simulink model "Verkehrspolizist"  (Simulink 8.7)
settings: Solver=FixedStepAuto  StartTime=0.0  StopTime=10.0  FixedStep=0.01  RelTol=1e-3
settings Model: Creator=eispin  LastModifiedBy=max
settings DataIOCC: LimitDataPoints=off  SaveFormat=Dataset
settings DebuggingCC: UnderspecifiedInitializationDetection=Simplified  MergeDetectMultiDrivingBlocksExec=error
settings HardwareCC: ProdBitPerPointer=64  ProdLargestAtomicFloat=Float  ProdIntDivRoundTo=Zero  ProdEndianess=LittleEndian  ProdWordSize=64  ProdHWDeviceType=Intel->x86-64 (Windows64)
settings ModelReferenceCC: PropagateSignalLabelsOutOfModel=on
settings ConfigComp: CovModelRefEnable=off

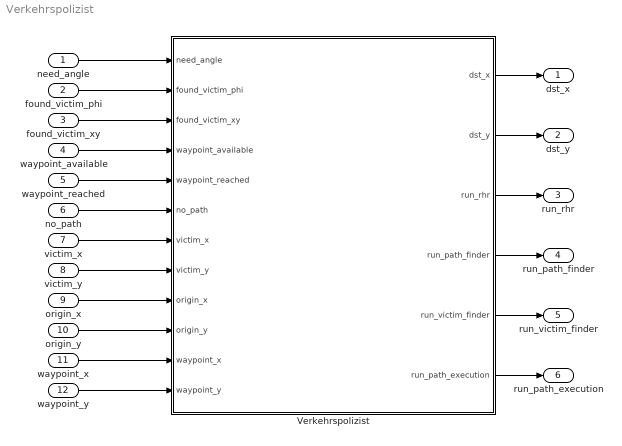
== system Verkehrspolizist ==
  need_angle : Inport
  found_victim_phi : Inport  Port=2
  found_victim_xy : Inport  Port=3
  waypoint_available : Inport  Port=4
  waypoint_reached : Inport  Port=5
  no_path : Inport  Port=6
  victim_x : Inport  Port=7
  victim_y : Inport  Port=8
  origin_x : Inport  Port=9
  origin_y : Inport  Port=10
  waypoint_x : Inport  Port=11
  waypoint_y : Inport  Port=12
  Verkehrspolizist : Stateflow chart  TreatAsAtomicUnit=on
  dst_x : Outport
  dst_y : Outport  Port=2
  run_rhr : Outport  Port=3
  run_path_finder : Outport  Port=4
  run_victim_finder : Outport  Port=5
  run_path_execution : Outport  Port=6
  wires:
  found_victim_phi/1 -> Verkehrspolizist/2(found_victim_phi)
  need_angle/1 -> Verkehrspolizist/1(need_angle)
  found_victim_xy/1 -> Verkehrspolizist/3(found_victim_xy)
  victim_x/1 -> Verkehrspolizist/7(victim_x)
  victim_y/1 -> Verkehrspolizist/8(victim_y)
  waypoint_available/1 -> Verkehrspolizist/4(waypoint_available)
  waypoint_reached/1 -> Verkehrspolizist/5(waypoint_reached)
  Verkehrspolizist/5(run_victim_finder) -> run_victim_finder/1
  Verkehrspolizist/4(run_path_finder) -> run_path_finder/1
  Verkehrspolizist/3(run_rhr) -> run_rhr/1
  Verkehrspolizist/2(dst_y) -> dst_y/1
  Verkehrspolizist/1(dst_x) -> dst_x/1
  waypoint_x/1 -> Verkehrspolizist/11(waypoint_x)
  waypoint_y/1 -> Verkehrspolizist/12(waypoint_y)
  origin_x/1 -> Verkehrspolizist/9(origin_x)
  origin_y/1 -> Verkehrspolizist/10(origin_y)
  no_path/1 -> Verkehrspolizist/6(no_path)
  Verkehrspolizist/6(run_path_execution) -> run_path_execution/1

== stateflow chart Verkehrspolizist ==
  state ExecutePath
    entry:
    run_path_finder = 0;
    run_path_execution = 1;
  state RoamTheStreetsToFindTracesOfVictim
    state Initialization
      entry:
      run_rhr = 1;
      run_path_finder = 0;
      run_victim_finder = 0;
      run_path_execution = 0;
    state GotVictimTrace
      % actually not needed, debugging only
      entry:
      run_victim_finder = 0;
      run_rhr = 1;
      exit:
      start_rescue = 1;
    (default) -> Initialization
    Initialization -> GotVictimTrace : [found_victim_phi == 1]
  state SenseAngle
    entry:
    run_rhr = 0;
    run_victim_finder = 1;
  state FollowPath
    state RunToVictim
      entry:
      run_rhr = 0;
      run_path_finder = 1;
      run_path_execution = 0;
      dst_x = victim_x;
      dst_y = victim_y;
    state GetOuttaHere
      % not needed, debugging/readability
      entry:
      run_path_finder = 1;
      run_path_execution = 0;
      dst_x = origin_x;
      dst_y = origin_y;
    (default) -> RunToVictim
    RunToVictim -> GetOuttaHere : [no_path = 1]
  state GetTheLadiesOrGentlemen
    % Done ^.^
  (default) -> RoamTheStreetsToFindTracesOfVictim
  RoamTheStreetsToFindTracesOfVictim -> SenseAngle [order 2] : [need_angle == 1]
  SenseAngle -> (history) : [found_victim_phi == 1]
  RoamTheStreetsToFindTracesOfVictim -> FollowPath [order 1] : [found_victim_phi == 1 && start_rescue == 1]
  FollowPath -> ExecutePath [order 1] : [waypoint_available == 1]
  ExecutePath -> (history) : [waypoint_reached == 1]
  FollowPath -> GetTheLadiesOrGentlemen [order 2] : [no_path == 1]
  data: need_angle input double; found_victim_phi input double; found_victim_xy input double; waypoint_available input double; waypoint_reached input double; no_path input double; victim_x input double; victim_y input double; origin_x input double; origin_y input double; dst_x output double; dst_y output double; run_rhr output double; run_path_finder output double; run_victim_finder output double; waypoint_x input double; waypoint_y input double; run_path_execution output double
